simulink model "Vehicle_Behavior_Modeling1"  (R2024b)
settings: Solver=FixedStepAuto  StartTime=0.0  StopTime=Inf  FixedStep=0.001  RelTol=1e-3
PostLoadFcn:
  | if any(exist('dsrtsu_mdlpostloadfcn', 'file') ~= 0), dsrtsu_mdlpostloadfcn('Execute', bdroot); end
InitFcn:
  | , if any(exist('rtifpga_mdlclblib', 'file') ~= 0), rtifpga_mdlclblib('Init', bdroot); end,
  | , if any(exist('dsmpb_private', 'file') ~= 0), dsmpb_private('dsmpb_mdlclblib', 'Init', bdroot); end,
model workspace (MAT data in the model file):
  indicator = -1
PreSaveFcn:
  | , if any(exist('dsmpb_private', 'file') ~= 0), dsmpb_private('dsmpb_mdlclblib', 'PreSave', bdroot); end,
CloseFcn:
  | , if any(exist('dsmpb_private', 'file') ~= 0), dsmpb_private('dsmpb_mdlclblib', 'Close', bdroot); end,
settings Model: DSMPB_ID_DATA={'833',struct('BlockId','6fc0dbc8-73ea-402d-818d-16f18e050b8c','SignalIds',{{'2b6451c0-fd0c-4268-8b2a-22dd17322f6d'}}),'834',struct('BlockId','7920a40d-cda9-4256-b1ac-2a33172fce8d','SignalIds',{{'35ea8044-d68c-4652-9a6a-3ae3cc9cc372'}}),'835',struct('BlockId','6449556e-3157-4f31-bd8d-aceb5faf945a','SignalIds',{{'ba591f74-be90-4468-9600-8bf28fcdd503'}}),'836',struct('BlockId','be469e62-25ec-4aaf-9adb-4878e55d3250','SignalIds',{{'bdb230ec-6523-429f-8dd6-6159c7d6bed7'}}),'837',struct('BlockId','b55725ac-9f2e-40a5-80c5-a3c6433921a7','SignalIds',{{'391bb536-a8a5-4602-8339-4d702f05ddac'}}),'838',struct('BlockId','12d7b802-2a0e-41ff-9011-d39c7a80f2ce','SignalIds',{{'65fa9323-a7aa-4c38-a564-149e867f53e8'}}),'839',struct('BlockId','b97fa48a-9fdc-42c7-be8b-2421995b9293','SignalIds',{{'f946b4af-18a3-4ff4-b560-56d5a56582a8'}}),'840',struct('BlockId','996af4dc-c5ca-433c-9fc9-66bd9ec8e223','SignalIds',{{'be412b3c-2616-4868-a31f-25495972eeb3'}})}  DSRTSU_INTERNAL_RTIFPGA=210  DSRTSU_INTERNAL_RTISTBM_VER=23.2  Creator=thipp  LastModifiedBy=MURTI
settings SolverCC: AutoInsertRateTranBlk=on
settings OptimizationCC: BlockReduction=off  ConditionallyExecuteInputs=off  OptimizeBlockIOStorage=off  BufferReuse=off  EnhancedBackFolding=on  PassReuseOutputArgsThreshold=0  MaxStackSize=64  OptimizeBlockOrder=speed  DifferentSizesBufferReuse=on
settings DebuggingCC: TasksWithSamePriorityMsg=none  ParameterTunabilityLossMsg=error
settings HardwareCC: ProdBitPerLong=64  ProdLargestAtomicInteger=Integer  ProdWordSize=32  ProdLongLongMode=on  ProdHWDeviceType=Custom Processor->Custom  UseEmbeddedCoderFeatures=off  UseSimulinkCoderFeatures=off
settings ModelReferenceCC: EnableParallelModelReferenceBuilds=on
settings SFSimCC: MATLABDynamicMemAlloc=off
settings RTWCC: Description=dSPACE Target DSRT - Generates SIC files for import by ConfigurationDesk and VEOS. Provides code generation for Simulink models imported in ConfigurationDesk.  SystemTargetFile=dsrt.tlc  GenCodeOnly=on  MakeCommand=make_dsrt  TemplateMakefile=dsrt_default_tmf  RTWVerbose=off  BuildConfiguration=Faster Runs
settings CodeAppCC: ForceParamTrailComments=on  OperatorAnnotations=on
settings STFCustomTargetCC: ParMdlRefBuildCompliant=on  SystemTargetFile=dsrt.tlc
settings GRTTargetCC: TargetLangStandard=C89/C90 (ANSI)  CompOptLevelCompliant=off  ConcurrentExecutionCompliant=off  CombineOutputUpdateFcns=off  MatFileLogging=off  CPPClassGenCompliant=off  UseToolchainInfoCompliant=off

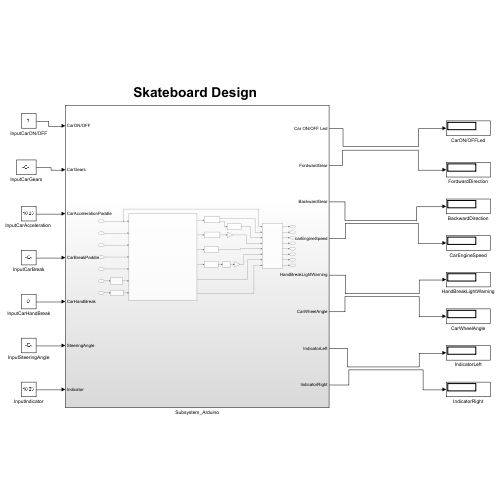
[thumbnail: Simulink's stored preview of the top-level diagram]
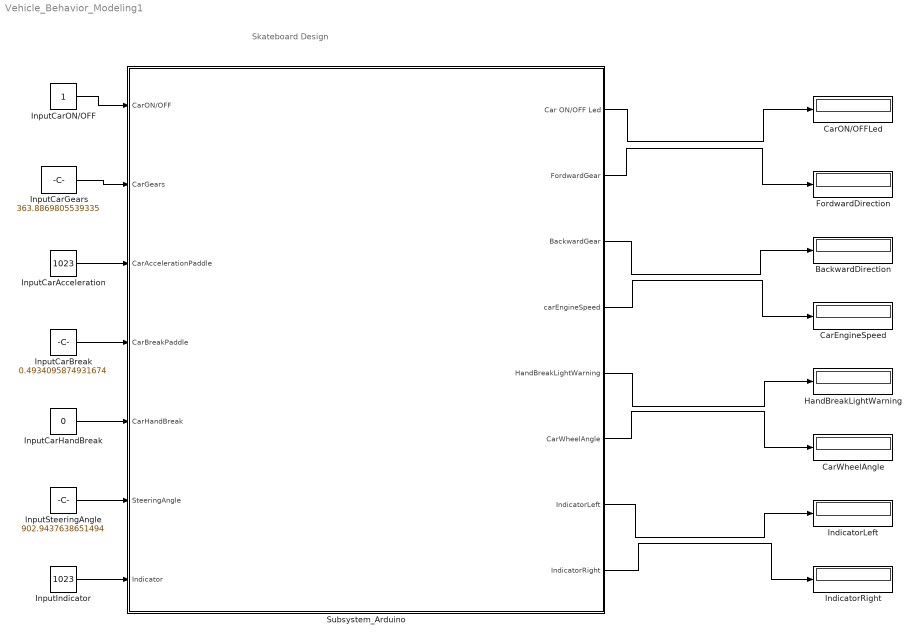
== system Vehicle_Behavior_Modeling1 ==
  note: Skateboard Design
  BackwardDirection : Display
  CarEngineSpeed : Display
  CarON/OFFLed : Display
  CarWheelAngle : Display
  FordwardDirection : Display
  HandBreakLightWarning : Display
  IndicatorLeft : Display
  IndicatorRight : Display
  "InputCarAcceleration " : Constant  Value=1023
  InputCarBreak : Constant  Value=0.4934095874931674
  InputCarGears : Constant  Value=363.8869805539335
  InputCarHandBreak : Constant  Value=0
  InputCarON/OFF : Constant
  InputIndicator : Constant  Value=1023
  InputSteeringAngle : Constant  Value=902.9437638651494
  Subsystem_Arduino : Subsystem
  wires:
  InputCarON/OFF/1 -> Subsystem_Arduino/1(CarON/OFF)
  Subsystem_Arduino/1(Car ON/OFF Led) -> CarON/OFFLed/1
  Subsystem_Arduino/4(carEngineSpeed) -> CarEngineSpeed/1
  "InputCarAcceleration "/1 -> Subsystem_Arduino/3(CarAccelerationPaddle)
  Subsystem_Arduino/7(IndicatorLeft) -> IndicatorLeft/1
  Subsystem_Arduino/6(CarWheelAngle) -> CarWheelAngle/1
  InputCarGears/1 -> Subsystem_Arduino/2(CarGears)
  Subsystem_Arduino/3(BackwardGear) -> BackwardDirection/1
  Subsystem_Arduino/2(FordwardGear) -> FordwardDirection/1
  InputIndicator/1 -> Subsystem_Arduino/7(Indicator)
  InputSteeringAngle/1 -> Subsystem_Arduino/6(SteeringAngle)
  InputCarHandBreak/1 -> Subsystem_Arduino/5("CarHandBreak ")
  Subsystem_Arduino/5(HandBreakLightWarning) -> HandBreakLightWarning/1
  Subsystem_Arduino/8(IndicatorRight) -> IndicatorRight/1
  InputCarBreak/1 -> Subsystem_Arduino/4(CarBreakPaddle)

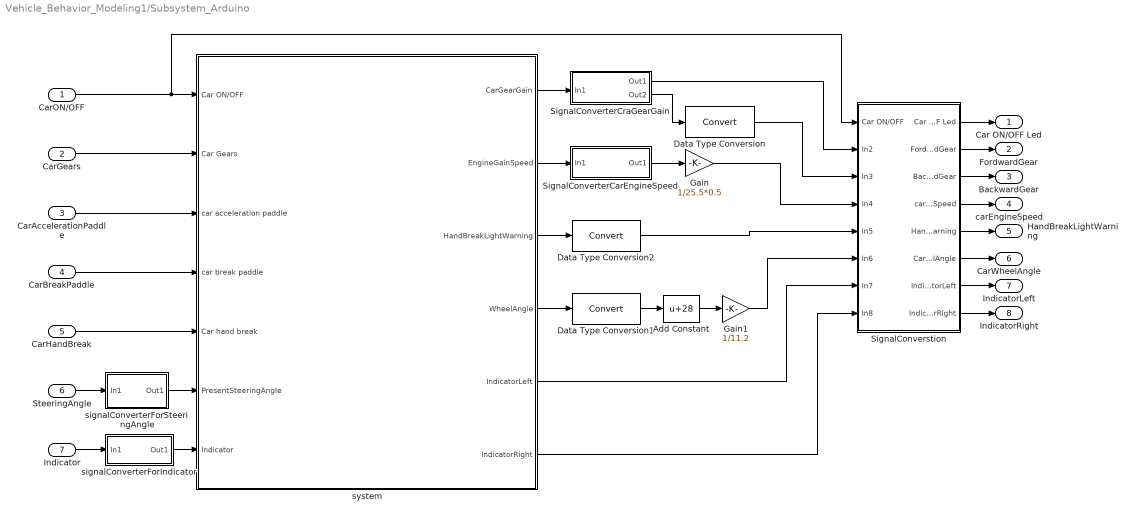
== system Vehicle_Behavior_Modeling1/Subsystem_Arduino ==
  CarON/OFF : Inport
  CarGears : Inport  Port=2
  CarAccelerationPaddle : Inport  Port=3
  CarBreakPaddle : Inport  Port=4
  "CarHandBreak " : Inport  Port=5
  SteeringAngle : Inport  Port=6
  Indicator : Inport  Port=7
  Add Constant : Bias  Bias=28  SaturateOnIntegerOverflow=off
  Data Type Conversion : DataTypeConversion  SaturateOnIntegerOverflow=off  RndMeth=Floor
  Data Type Conversion1 : DataTypeConversion  SaturateOnIntegerOverflow=off  RndMeth=Floor
  Data Type Conversion2 : DataTypeConversion  SaturateOnIntegerOverflow=off  RndMeth=Floor
  Gain : Gain  Gain=1/25.5*0.5
  Gain1 : Gain  Gain=1/11.2
  SignalConverstion : Subsystem
  SignalConverterCarEngineSpeed : Subsystem
  SignalConverterCraGearGain : Subsystem
  signalConverterForIndicator : Subsystem
  signalConverterForSteeringAngle : Subsystem
  system : Subsystem
  Car ON/OFF Led : Outport
  FordwardGear : Outport  Port=2
  BackwardGear : Outport  Port=3
  carEngineSpeed : Outport  Port=4
  HandBreakLightWarning : Outport  Port=5
  CarWheelAngle : Outport  Port=6
  IndicatorLeft : Outport  Port=7
  IndicatorRight : Outport  Port=8
  wires:
  CarBreakPaddle/1 -> system/4(car break paddle)
  CarAccelerationPaddle/1 -> system/3(car acceleration paddle)
  "CarHandBreak "/1 -> system/5("Car hand break ")
  CarGears/1 -> system/2(Car Gears)
  CarON/OFF/1 -> SignalConverstion/1(Car ON/OFF), system/1(Car ON/OFF)
  SteeringAngle/1 -> signalConverterForSteeringAngle/1(In1)
  signalConverterForSteeringAngle/1(Out1) -> system/6(PresentSteeringAngle)
  Indicator/1 -> signalConverterForIndicator/1(In1)
  signalConverterForIndicator/1(Out1) -> system/7(Indicator)
  system/2(EngineGainSpeed) -> SignalConverterCarEngineSpeed/1(In1)
  system/1(CarGearGain) -> SignalConverterCraGearGain/1(In1)
  SignalConverterCraGearGain/2(Out2) -> Data Type Conversion/1
  system/4(WheelAngle) -> Data Type Conversion1/1
  system/3(HandBreakLightWarning) -> Data Type Conversion2/1
  SignalConverterCarEngineSpeed/1(Out1) -> Gain/1
  Data Type Conversion1/1 -> Add Constant/1
  Add Constant/1 -> Gain1/1
  Data Type Conversion/1 -> SignalConverstion/3(In3)
  Gain/1 -> SignalConverstion/4(In4)
  Data Type Conversion2/1 -> SignalConverstion/5(In5)
  Gain1/1 -> SignalConverstion/6(In6)
  system/5(IndicatorLeft) -> SignalConverstion/7(In7)
  system/6(IndicatorRight) -> SignalConverstion/8(In8)
  SignalConverstion/1(Car ON/OFF Led) -> Car ON/OFF Led/1
  SignalConverstion/2(FordwardGear) -> FordwardGear/1
  SignalConverstion/3(BackwardGear) -> BackwardGear/1
  SignalConverstion/4(carEngineSpeed) -> carEngineSpeed/1
  SignalConverstion/5(HandBreakLightWarning) -> HandBreakLightWarning/1
  SignalConverstion/6(CarWheelAngle) -> CarWheelAngle/1
  SignalConverstion/7(IndicatorLeft) -> IndicatorLeft/1
  SignalConverstion/8(IndicatorRight) -> IndicatorRight/1
  SignalConverterCraGearGain/1(Out1) -> SignalConverstion/2(In2)

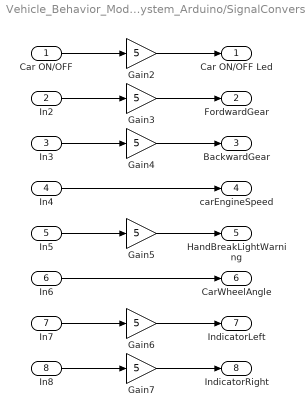
== system Vehicle_Behavior_Modeling1/Subsystem_Arduino/SignalConverstion ==
  Car ON/OFF : Inport
  In2 : Inport  Port=2
  In3 : Inport  Port=3
  In4 : Inport  Port=4
  In5 : Inport  Port=5
  In6 : Inport  Port=6
  In7 : Inport  Port=7
  In8 : Inport  Port=8
  Gain{2..7} (6 alike) : Gain  Gain=5
  Car ON/OFF Led : Outport
  FordwardGear : Outport  Port=2
  BackwardGear : Outport  Port=3
  carEngineSpeed : Outport  Port=4
  HandBreakLightWarning : Outport  Port=5
  CarWheelAngle : Outport  Port=6
  IndicatorLeft : Outport  Port=7
  IndicatorRight : Outport  Port=8
  wires:
  In6/1 -> CarWheelAngle/1
  In4/1 -> carEngineSpeed/1
  Gain3/1 -> FordwardGear/1
  Gain7/1 -> IndicatorRight/1
  Gain5/1 -> HandBreakLightWarning/1
  In5/1 -> Gain5/1
  Gain4/1 -> BackwardGear/1
  Gain6/1 -> IndicatorLeft/1
  Gain2/1 -> Car ON/OFF Led/1
  In3/1 -> Gain4/1
  In7/1 -> Gain6/1
  In8/1 -> Gain7/1
  In2/1 -> Gain3/1
  Car ON/OFF/1 -> Gain2/1

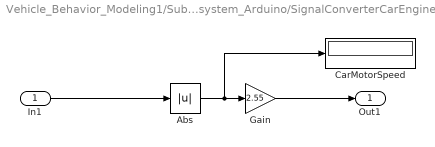
== system Vehicle_Behavior_Modeling1/Subsystem_Arduino/SignalConverterCarEngineSpeed ==
  In1 : Inport
  Abs : Abs  SaturateOnIntegerOverflow=off
  CarMotorSpeed : Display
  Gain : Gain  Gain=2.55
  Out1 : Outport
  wires:
  Abs/1 -> CarMotorSpeed/1, Gain/1
  Gain/1 -> Out1/1
  In1/1 -> Abs/1

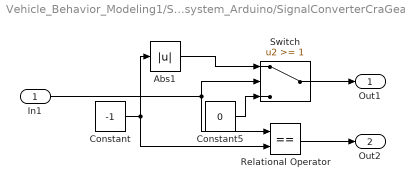
== system Vehicle_Behavior_Modeling1/Subsystem_Arduino/SignalConverterCraGearGain ==
  In1 : Inport
  Abs1 : Abs  SaturateOnIntegerOverflow=off
  Constant : Constant  Value=-1
  Constant5 : Constant  Value=0
  Relational Operator : RelationalOperator  Operator===  OutDataTypeStr=boolean  RndMeth=Simplest  InputSameDT=off
  Switch : Switch  Threshold=1  SaturateOnIntegerOverflow=off  InputSameDT=off
  Out1 : Outport
  Out2 : Outport  Port=2
  wires:
  Switch/1 -> Out1/1
  Abs1/1 -> Switch/1
  Constant5/1 -> Switch/3
  Constant/1 -> Relational Operator/2, Abs1/1
  In1/1 -> Relational Operator/1, Switch/2
  Relational Operator/1 -> Out2/1

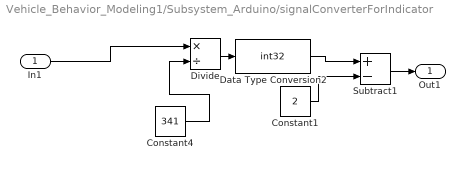
== system Vehicle_Behavior_Modeling1/Subsystem_Arduino/signalConverterForIndicator ==
  In1 : Inport
  Constant1 : Constant  Value=2
  Constant4 : Constant  Value=341
  Data Type Conversion2 : DataTypeConversion  OutDataTypeStr=int32  ConvertRealWorld=Stored Integer (SI)  RndMeth=Ceiling  SaturateOnIntegerOverflow=off
  Divide : Product  Inputs=*/
  Subtract1 : Sum  Inputs=+-
  Out1 : Outport
  wires:
  Constant4/1 -> Divide/2
  Data Type Conversion2/1 -> Subtract1/1
  Divide/1 -> Data Type Conversion2/1
  Subtract1/1 -> Out1/1
  Constant1/1 -> Subtract1/2
  In1/1 -> Divide/1

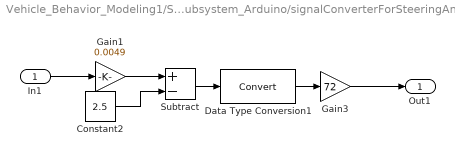
== system Vehicle_Behavior_Modeling1/Subsystem_Arduino/signalConverterForSteeringAngle ==
  In1 : Inport
  Constant2 : Constant  Value=2.5
  Data Type Conversion1 : DataTypeConversion  SaturateOnIntegerOverflow=off  RndMeth=Floor
  Gain1 : Gain  Gain=0.0049
  Gain3 : Gain  Gain=72
  Subtract : Sum  Inputs=+-
  Out1 : Outport
  wires:
  Gain1/1 -> Subtract/1
  Constant2/1 -> Subtract/2
  Subtract/1 -> Data Type Conversion1/1
  Gain3/1 -> Out1/1
  In1/1 -> Gain1/1
  Data Type Conversion1/1 -> Gain3/1

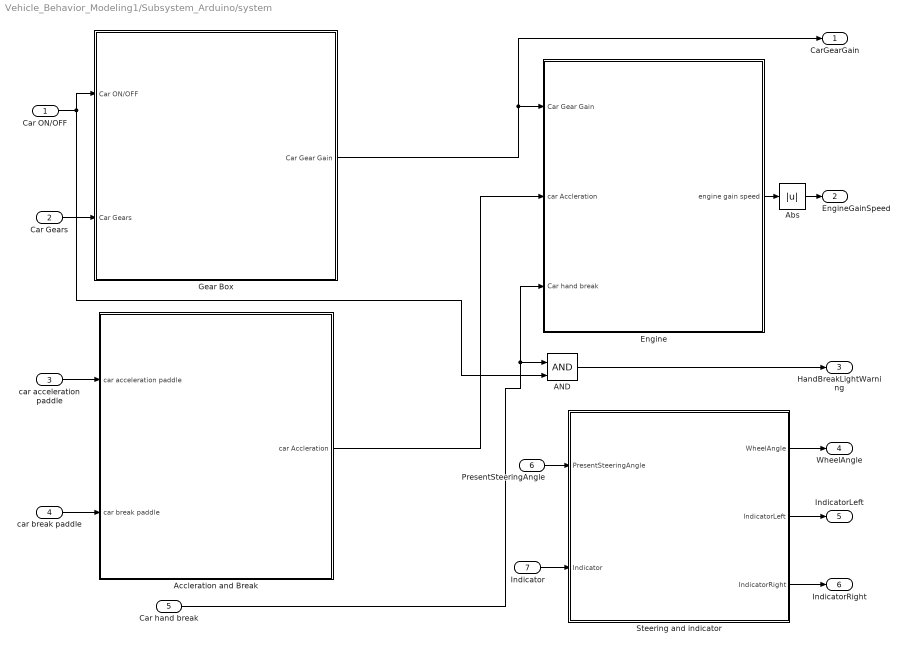
== system Vehicle_Behavior_Modeling1/Subsystem_Arduino/system ==
  Car ON/OFF : Inport
  Car Gears : Inport  Port=2
  car acceleration paddle : Inport  Port=3
  car break paddle : Inport  Port=4
  "Car hand break " : Inport  Port=5
  PresentSteeringAngle : Inport  Port=6
  Indicator : Inport  Port=7
  AND : Logic  IconShape=distinctive  AllPortsSameDT=off  OutDataTypeStr=boolean
  Abs : Abs  SaturateOnIntegerOverflow=off
  Accleration and Break : Subsystem
  Engine : Subsystem
  Gear Box : Subsystem
  "Steering and indicator " : Subsystem
  CarGearGain : Outport
  EngineGainSpeed : Outport  Port=2
  HandBreakLightWarning : Outport  Port=3
  WheelAngle : Outport  Port=4
  IndicatorLeft : Outport  Port=5
  IndicatorRight : Outport  Port=6
  wires:
  Car ON/OFF/1 -> Gear Box/1(Car ON/OFF), AND/2
  Accleration and Break/1(car Accleration) -> Engine/2(car Accleration)
  "Steering and indicator "/3(IndicatorRight) -> IndicatorRight/1
  "Steering and indicator "/2(IndicatorLeft) -> IndicatorLeft/1
  car acceleration paddle/1 -> Accleration and Break/1(car acceleration paddle)
  Indicator/1 -> "Steering and indicator "/2(Indicator)
  "Car hand break "/1 -> Engine/3("Car hand break "), AND/1
  Engine/1(engine gain speed) -> Abs/1
  car break paddle/1 -> Accleration and Break/2(car break paddle)
  Car Gears/1 -> Gear Box/2(Car Gears)
  Abs/1 -> EngineGainSpeed/1
  "Steering and indicator "/1(WheelAngle) -> WheelAngle/1
  AND/1 -> HandBreakLightWarning/1
  PresentSteeringAngle/1 -> "Steering and indicator "/1(PresentSteeringAngle)
  Gear Box/1(Car Gear Gain) -> CarGearGain/1, Engine/1(Car Gear Gain)

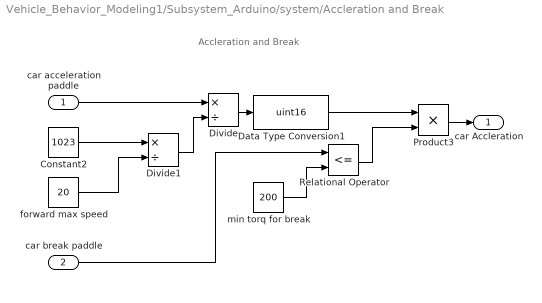
== system Vehicle_Behavior_Modeling1/Subsystem_Arduino/system/Accleration and Break ==
  note: Accleration and Break
  car acceleration paddle : Inport
  car break paddle : Inport  Port=2
  Constant2 : Constant  Value=1023
  Data Type Conversion1 : DataTypeConversion  OutDataTypeStr=uint16  SaturateOnIntegerOverflow=off  RndMeth=Floor
  Divide : Product  Inputs=*/  RndMeth=Zero  SaturateOnIntegerOverflow=on
  Divide1 : Product  Inputs=*/  RndMeth=Zero  SaturateOnIntegerOverflow=on
  Product3 : Product
  Relational Operator : RelationalOperator  Operator=<=  OutDataTypeStr=boolean  RndMeth=Simplest  InputSameDT=off
  forward max speed : Constant  Value=20
  min torq for break : Constant  Value=200
  car Accleration : Outport
  wires:
  min torq for break/1 -> Relational Operator/2
  Divide/1 -> Data Type Conversion1/1
  forward max speed/1 -> Divide1/2
  car break paddle/1 -> Relational Operator/1
  Data Type Conversion1/1 -> Product3/1
  Constant2/1 -> Divide1/1
  Divide1/1 -> Divide/2
  Relational Operator/1 -> Product3/2
  car acceleration paddle/1 -> Divide/1
  Product3/1 -> car Accleration/1

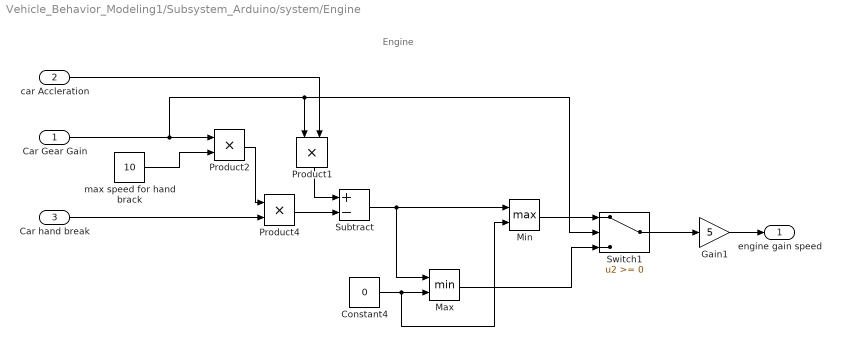
== system Vehicle_Behavior_Modeling1/Subsystem_Arduino/system/Engine ==
  note: Engine
  Car Gear Gain : Inport
  car Accleration : Inport  Port=2
  "Car hand break " : Inport  Port=3
  Constant4 : Constant  Value=0
  Gain1 : Gain  Gain=5
  Max : MinMax  Inputs=2
  Min : MinMax  Function=max  Inputs=2
  Product1 : Product
  Product2 : Product
  Product4 : Product
  Subtract : Sum  Inputs=+-
  Switch1 : Switch  SaturateOnIntegerOverflow=off  InputSameDT=off
  max speed for hand brack : Constant  Value=10
  engine gain speed : Outport
  wires:
  Subtract/1 -> Min/1, Max/1
  Switch1/1 -> Gain1/1
  Product2/1 -> Product4/1
  Product1/1 -> Subtract/1
  Product4/1 -> Subtract/2
  Constant4/1 -> Min/2, Max/2
  max speed for hand brack/1 -> Product2/2
  Car Gear Gain/1 -> Product1/1, Switch1/2, Product2/1
  Max/1 -> Switch1/3
  Min/1 -> Switch1/1
  car Accleration/1 -> Product1/2
  "Car hand break "/1 -> Product4/2
  Gain1/1 -> engine gain speed/1

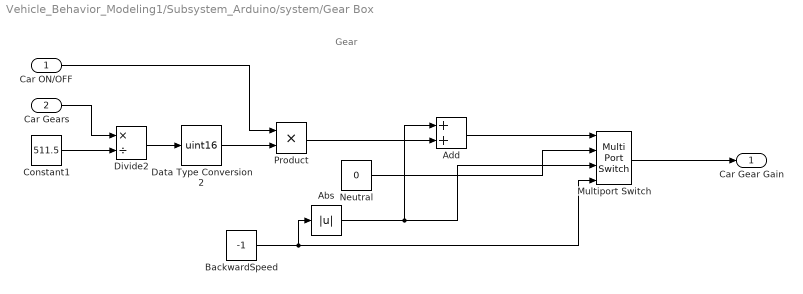
== system Vehicle_Behavior_Modeling1/Subsystem_Arduino/system/Gear Box ==
  note: Gear
  Car ON/OFF : Inport
  Car Gears : Inport  Port=2
  Abs : Abs  SaturateOnIntegerOverflow=off
  Add : Sum
  BackwardSpeed : Constant  Value=-1
  Constant1 : Constant  Value=511.5
  Data Type Conversion2 : DataTypeConversion  OutDataTypeStr=uint16  RndMeth=Nearest  SaturateOnIntegerOverflow=off
  Divide2 : Product  Inputs=*/  RndMeth=Zero  SaturateOnIntegerOverflow=on
  Multiport Switch : MultiPortSwitch  SaturateOnIntegerOverflow=off  InputSameDT=off
  Neutral : Constant  Value=0
  Product : Product
  Car Gear Gain : Outport
  wires:
  Add/1 -> Multiport Switch/1
  Neutral/1 -> Multiport Switch/2
  Constant1/1 -> Divide2/2
  Product/1 -> Add/2
  BackwardSpeed/1 -> Abs/1, Multiport Switch/4
  Data Type Conversion2/1 -> Product/2
  Divide2/1 -> Data Type Conversion2/1
  Abs/1 -> Add/1, Multiport Switch/3
  Multiport Switch/1 -> Car Gear Gain/1
  Car ON/OFF/1 -> Product/1
  Car Gears/1 -> Divide2/1

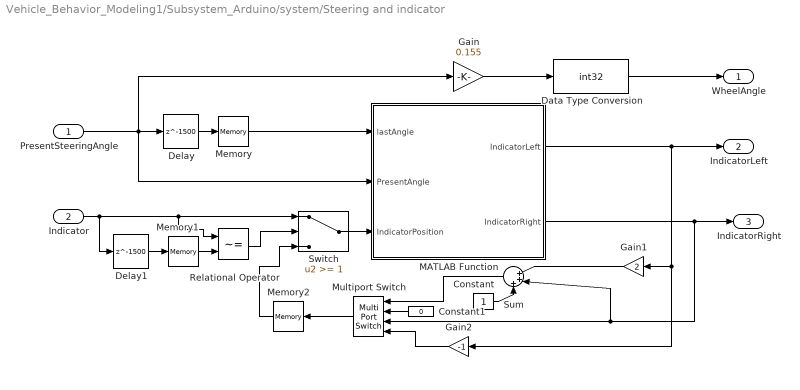
== system Vehicle_Behavior_Modeling1/Subsystem_Arduino/system/Steering and indicator  ==
  PresentSteeringAngle : Inport
  Indicator : Inport  Port=2
  Constant : Constant
  Constant1 : Constant  Value=0
  Data Type Conversion : DataTypeConversion  OutDataTypeStr=int32  SaturateOnIntegerOverflow=off  RndMeth=Floor
  Delay : Delay  DelayLength=1500
  Delay1 : Delay  DelayLength=1500
  Gain : Gain  Gain=0.155
  Gain1 : Gain  Gain=2
  Gain2 : Gain  Gain=-1
  MATLAB Function : MATLAB Function  TreatAsAtomicUnit=on
  Memory : Memory
  Memory1 : Memory
  Memory2 : Memory
  Multiport Switch : MultiPortSwitch  SaturateOnIntegerOverflow=off  InputSameDT=off
  Relational Operator : RelationalOperator  Operator=~=  OutDataTypeStr=boolean  RndMeth=Simplest  InputSameDT=off
  Sum : Sum  Inputs=|+++
  Switch : Switch  Threshold=1  SaturateOnIntegerOverflow=off  InputSameDT=off
  WheelAngle : Outport
  IndicatorLeft : Outport  Port=2
  IndicatorRight : Outport  Port=3
  wires:
  PresentSteeringAngle/1 -> MATLAB Function/2(PresentAngle), Gain/1, Delay/1
  MATLAB Function/1(IndicatorLeft) -> Gain2/1, Gain1/1, IndicatorLeft/1
  Memory/1 -> MATLAB Function/1(lastAngle)
  Delay/1 -> Memory/1
  Indicator/1 -> Delay1/1, Relational Operator/1, Switch/1
  Relational Operator/1 -> Switch/2
  Switch/1 -> MATLAB Function/3(IndicatorPosition)
  Memory1/1 -> Relational Operator/2
  Delay1/1 -> Memory1/1
  Memory2/1 -> Switch/3
  Sum/1 -> Multiport Switch/1
  Constant/1 -> Sum/3
  Constant1/1 -> Multiport Switch/2
  MATLAB Function/2(IndicatorRight) -> IndicatorRight/1, Sum/2, Multiport Switch/3
  Gain1/1 -> Sum/1
  Gain2/1 -> Multiport Switch/4
  Multiport Switch/1 -> Memory2/1
  Gain/1 -> Data Type Conversion/1
  Data Type Conversion/1 -> WheelAngle/1

== matlab function Vehicle_Behavior_Modeling1/Subsystem_Arduino/system/Steering and indicator /MATLAB Function ==
  data: IndicatorLeft output; IndicatorRight output; lastAngle input; PresentAngle input; IndicatorPosition input
function [IndicatorLeft, IndicatorRight] = fcn(lastAngle, PresentAngle, IndicatorPosition)
    % Determine the turning direction
    turning = 0;
    if PresentAngle> lastAngle 
        turning = 1; % Turning right
    elseif PresentAngle< lastAngle 
        turning = -1; % Turning left
    end
    
    % Update the indicator position based on the turning direction
    if IndicatorPosition == 1 && turning == -1
        IndicatorPosition = 0; % Cancel right indicator when turning left
    elseif IndicatorPosition == -1 && turning == 1
        IndicatorPosition = 0; % Cancel left indicator when turning right
    end
    
    % Determine the state of left and right indicators
    if IndicatorPosition == -1
        IndicatorLeft = 1; % Left indicator is on
    else
        IndicatorLeft = 0;
    end
    if IndicatorPosition == 1
        IndicatorRight = 1; % Right indicator is on
    else
        IndicatorRight = 0;
    end
end
